simulink model "Radar_MTI"  (R2024a)
settings: Solver=FixedStepDiscrete  StartTime=0.0  StopTime=0.03  FixedStep=0.00002  RelTol=1e-3
libraries: dspxfrm3 x1, dspsrcs4 x1
settings Model: Creator=pc  LastModifiedBy=pc

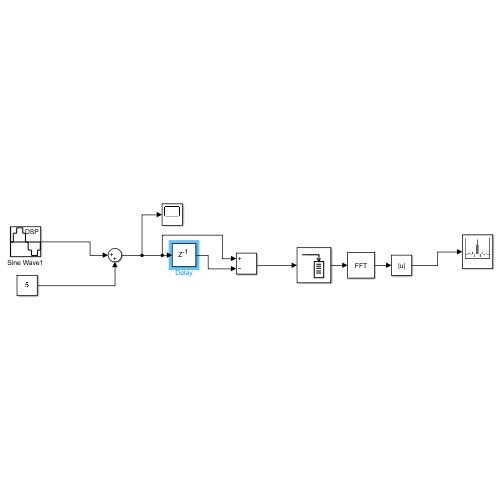
[thumbnail: Simulink's stored preview of the top-level diagram]
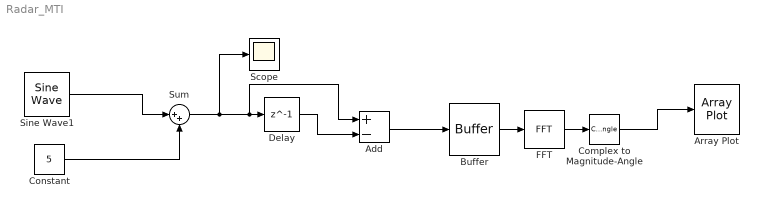
== system Radar_MTI ==
  Add : Sum  Inputs=+-
  Array Plot : ArrayPlot  WindowPosition=[796.000000,133.000000,560.000000,408.000000,]  Visible=on  ScopeFrameLocation=window  YLimits=[-93.5693 93.5693]
  Buffer : Buffer  N=128  OutputFrames=off
  Complex to Magnitude-Angle : ComplexToMagnitudeAngle  Output=Magnitude
  Constant : Constant  Value=5  SampleTime=0.00002
  Delay : Delay  DelayLength=1  InitialCondition=0  SampleTime=0.00002
  FFT : dspxfrm3/FFT  FFTImplementation=Auto  CompMethod=Table lookup  TableOpt=NEW  TableOptActive=Speed  BitRevOrder=off  Normalize=off  InheritFFTLength=off  FFTLength=128  WrapInput=off  roundingMode=Ceiling  overflowMode=off  firstCoeffDataTypeStr=Inherit: Same word length as input  firstCoeffLastDataTypeStr=Inherit: Same word length as input  outputMin=[]  outputMax=[]
  Scope : Scope
  Sine Wave1 : dspsrcs4/Sine Wave  Amplitude=1  Frequency=16666  Phase=0  SampleMode=Discrete  OutComplex=Real  CompMethod=Trigonometric fcn  TableSize=Speed  SampleTime=0.00002  SamplesPerFrame=1  ResetState=Restart at time zero  OutputFrames=off  dataType=double  wordLen=16  udDataType=sfix(16)  fracBitsMode=Best precision  numFracBits=15  OutDataTypeStr=double  LastOutDataTypeStr=double
  Sum : Sum  Inputs=|++
  wires:
  Sine Wave1/1 -> Sum/1
  Constant/1 -> Sum/2
  Sum/1 -> Scope/1, Add/1, Delay/1
  Delay/1 -> Add/2
  Add/1 -> Buffer/1
  Buffer/1 -> FFT/1
  FFT/1 -> Complex to Magnitude-Angle/1
  Complex to Magnitude-Angle/1 -> Array Plot/1
